simulink model "sistema_completo_con_controlador_pid_no_ideal"  (R2019a)
settings: Solver=VariableStepAuto  StartTime=0.0  StopTime=25  MaxStep=1e-5  RelTol=1e-5
undefined symbols (not defined in the file): A_sensor_curr, A_sensor_pos, A_sensor_temp, alpha_cu, b_eq, B_sensor_curr, B_sensor_pos, B_sensor_temp, C_sensor_curr, C_sensor_pos, C_sensor_temp, C_ts, D_sensor_curr, D_sensor_pos, D_sensor_temp, dT_l, J_eq, K_d, K_i, K_p, Ke_theta, Ke_w, L_d, L_ls, L_q, lambda_m, P_p, r, R_0, R_d, R_q, R_s_40, R_ts_amb, t_high, t_rise, w_max
libraries: eeTransforms x5, simulink x3
settings Model: Creator=pedro  LastModifiedBy=pedro

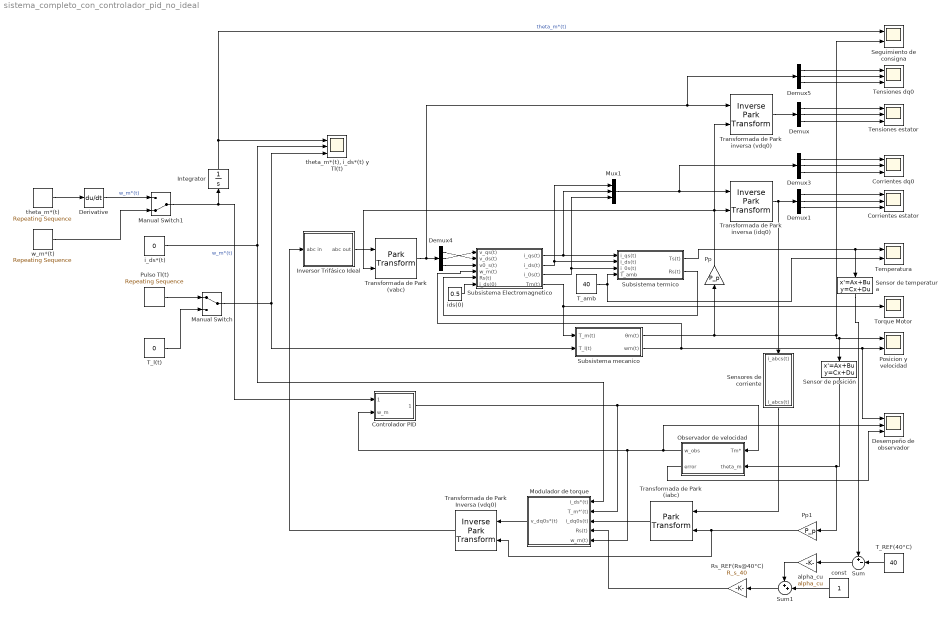
== system sistema_completo_con_controlador_pid_no_ideal ==
  " theta_m*(t), i_ds*(t) y Tl(t)" : Scope  NumInputPorts=3
  Controlador PID : Subsystem
  Corrientes estator : Scope  NumInputPorts=3
  Corrientes dq0 : Scope  NumInputPorts=3
  Demux{,1,3..5} (5 alike) : Demux  Outputs=3
  Derivative : Derivative
  Desempeño de observador : Scope  NumInputPorts=3
  Integrator : Integrator
  Inversor Trifásico Ideal : Subsystem
  Manual Switch : ManualSwitch
  Manual Switch1 : ManualSwitch  CurrentSetting=0
  Modulador de torque : Subsystem
  Mux1 : Mux  Inputs=3
  Observador de velocidad : Subsystem
  Posicion y velocidad : Scope  NumInputPorts=2
  Pp : Gain  Gain=P_p
  Pp1 : Gain  Gain=P_p
  Pulso Tl(t) : simulink/Sources/Repeating Sequence  rep_seq_t=[0 2.99 3 6.99 7 13.99 14 15.99 16 25]  rep_seq_y=[0 0 dT_l dT_l 0 0 -dT_l -dT_l 0 0]
  Rs_REF(Rs@40°C) : Gain  Gain=R_s_40
  Seguimiento de consigna : Scope  NumInputPorts=2
  Sensor de posición : StateSpace  A=A_sensor_pos  B=B_sensor_pos  C=C_sensor_pos  D=D_sensor_pos  InitialCondition=0  ContinuousStateAttributes="\"position\""
  Sensor de temperatura : StateSpace  A=A_sensor_temp  B=B_sensor_temp  C=C_sensor_temp  D=D_sensor_temp  InitialCondition=0  ContinuousStateAttributes="\"temperature\""
  Sensores de corriente : Subsystem
  Subsistema Electromagnetico : Subsystem
  "Subsistema mecanico " : Subsystem
  "Subsistema termico " : Subsystem
  Sum : Sum  Inputs=+-|
  Sum1 : Sum  Inputs=++|
  T_REF(40°C) : Constant  Value=40
  T_amb : Constant  Value=40
  T_l(t) : Constant  Value=0
  Temperatura : Scope  NumInputPorts=2
  Tensiones estator : Scope  NumInputPorts=3
  Tensiones dq0 : Scope  NumInputPorts=3
  Torque Motor : Scope
  Transformada de Park (iabc) : eeTransforms/Park Transform  AxisAlignment=Q-axis  PowerInvariant=off
      settings: SourceProductName=Simscape Electrical
  "Transformada de Park (vabc) " : eeTransforms/Park Transform  AxisAlignment=Q-axis  PowerInvariant=off
      settings: SourceProductName=Simscape Electrical
  Transformada de Park Inversa (vdq0) : eeTransforms/Inverse Park Transform  AxisAlignment=Q-axis  PowerInvariant=off
      settings: SourceProductName=Simscape Electrical
  Transformada de Park inversa (idq0) : eeTransforms/Inverse Park Transform  AxisAlignment=Q-axis  PowerInvariant=off
      settings: SourceProductName=Simscape Electrical
  "Transformada de Park inversa (vdq0) " : eeTransforms/Inverse Park Transform  AxisAlignment=Q-axis  PowerInvariant=off
      settings: SourceProductName=Simscape Electrical
  alpha_cu : Gain  Gain=alpha_cu
  const : Constant
  i_ds*(t) : Constant  Value=0
  ids(0) : Constant  Value=0.5
  theta_m*(t) : simulink/Sources/Repeating Sequence  rep_seq_t=[0 5 10 15 20 25]  rep_seq_y=[0 0 2*r*pi 2*r*pi 0 0]
  w_m*(t) : simulink/Sources/Repeating Sequence  rep_seq_t=[0 5 (5+t_rise) (5+t_rise+t_high) (5+2*t_rise+t_high) 15 (15+t_rise) (15+t_rise+t_high) (15+2*t_rise+t_high) 25]  rep_seq_y=[0 0 w_max w_max 0 0 -w_max -w_max 0 0]
  wires:
  Subsistema Electromagnetico/1("i_qs(t) ") -> Mux1/2, "Subsistema termico "/1("i_qs(t) ")
  Pp1/1 -> Transformada de Park Inversa (vdq0)/2, Transformada de Park (iabc)/2
  ids(0)/1 -> Subsistema Electromagnetico/6(i_ds(0))
  Demux/1 -> Tensiones estator/1
  Demux3/2 -> Corrientes dq0/2
  Transformada de Park inversa (idq0)/1 -> Demux1/1, Sensores de corriente/1(i_abcs(t))
  Sensores de corriente/1("i_abcs(t) ") -> Transformada de Park (iabc)/1
  Demux1/3 -> Corrientes estator/3
  Demux5/2 -> Tensiones dq0/2
  Demux/3 -> Tensiones estator/3
  Demux5/3 -> Tensiones dq0/3
  Demux/2 -> Tensiones estator/2
  Demux4/3 -> Subsistema Electromagnetico/3(v0_s(t))
  Inversor Trifásico Ideal/1(abc out) -> "Transformada de Park (vabc) "/1
  "Subsistema termico "/2(Rs(t)) -> Subsistema Electromagnetico/5("Rs(t) ")
  Pp/1 -> "Transformada de Park (vabc) "/2, Transformada de Park inversa (idq0)/2, "Transformada de Park inversa (vdq0) "/2
  Manual Switch/1 -> " theta_m*(t), i_ds*(t) y Tl(t)"/3, "Subsistema mecanico "/2("T_l(t) ")
  Demux1/2 -> Corrientes estator/2
  Demux4/2 -> Subsistema Electromagnetico/1(v_qs(t))
  Subsistema Electromagnetico/3("i_0s(t) ") -> Mux1/3, "Subsistema termico "/3(i_0s(t))
  "Transformada de Park inversa (vdq0) "/1 -> Demux/1
  Demux4/1 -> Subsistema Electromagnetico/2(v_ds(t))
  T_amb/1 -> Temperatura/2, "Subsistema termico "/4(T_amb)
  Demux1/1 -> Corrientes estator/1
  "Transformada de Park (vabc) "/1 -> Demux5/1, "Transformada de Park inversa (vdq0) "/1, Demux4/1
  Demux5/1 -> Tensiones dq0/1
  Transformada de Park (iabc)/1 -> Modulador de torque/3(i_dq0s(t))
  Demux3/3 -> Corrientes dq0/3
  Demux3/1 -> Corrientes dq0/1
  Mux1/1 -> Transformada de Park inversa (idq0)/1, Demux3/1
  Subsistema Electromagnetico/2(i_ds(t)) -> Mux1/1, "Subsistema termico "/2("i_ds(t) ")
  "Subsistema mecanico "/2(wm(t)) -> Posicion y velocidad/2, Desempeño de observador/1, Subsistema Electromagnetico/4(w_m(t))
  "Subsistema mecanico "/1(θm(t)) -> Sensor de posición/1, Posicion y velocidad/1, Seguimiento de consigna/2, Pp/1
  Subsistema Electromagnetico/4(Tm(t)) -> "Subsistema mecanico "/1("T_m(t) "), Torque Motor/1
  "Subsistema termico "/1(Ts(t)) -> Temperatura/1, Sensor de temperatura/1
  Sensor de posición/1 -> Pp1/1, Observador de velocidad/2(theta_m)
  Transformada de Park Inversa (vdq0)/1 -> Inversor Trifásico Ideal/1(abc in)
  i_ds*(t)/1 -> Modulador de torque/1(i_ds*(t)), " theta_m*(t), i_ds*(t) y Tl(t)"/2
  Observador de velocidad/1(w_obs) -> Desempeño de observador/2, Modulador de torque/5(w_m(t)), Controlador PID/2(w_m)
  Controlador PID/1(T_m*'(t)) -> Modulador de torque/2(T_m*'(t)), Observador de velocidad/1(Tm*)
  Modulador de torque/1(v_dq0s*(t)) -> Transformada de Park Inversa (vdq0)/1
  theta_m*(t)/1 -> Derivative/1
  Manual Switch1/1 -> Integrator/1, Controlador PID/1(w_m*)  "w_m*(t)"
  Observador de velocidad/2(error) -> Desempeño de observador/3
  Pulso Tl(t)/1 -> Manual Switch/1
  T_l(t)/1 -> Manual Switch/2
  Derivative/1 -> Manual Switch1/1  "w_m*(t)"
  Integrator/1 -> " theta_m*(t), i_ds*(t) y Tl(t)"/1, Seguimiento de consigna/1  "theta_m*(t)"
  w_m*(t)/1 -> Manual Switch1/2
  Sum/1 -> alpha_cu/1
  alpha_cu/1 -> Sum1/1
  Sum1/1 -> Rs_REF(Rs@40°C)/1
  const/1 -> Sum1/2
  T_REF(40°C)/1 -> Sum/2
  Sensor de temperatura/1 -> Sum/1
  Rs_REF(Rs@40°C)/1 -> Modulador de torque/4(Rs(t))

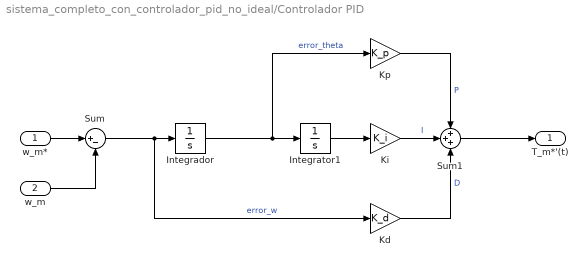
== system sistema_completo_con_controlador_pid_no_ideal/Controlador PID ==
  w_m* : Inport
  w_m : Inport  Port=2
  Integrador : Integrator
  Integrator1 : Integrator
  Kd : Gain  Gain=K_d
  Ki : Gain  Gain=K_i
  Kp : Gain  Gain=K_p
  Sum : Sum  Inputs=|+-
  Sum1 : Sum  Inputs=+++
  T_m*'(t) : Outport
  wires:
  Sum/1 -> Kd/1, Integrador/1  "error_w"
  w_m/1 -> Sum/2
  Sum1/1 -> T_m*'(t)/1
  Integrador/1 -> Integrator1/1, Kp/1  "error_theta"
  Kd/1 -> Sum1/3  "D"
  Integrator1/1 -> Ki/1
  w_m*/1 -> Sum/1
  Ki/1 -> Sum1/2  "I"
  Kp/1 -> Sum1/1  "P"

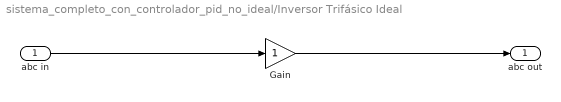
== system sistema_completo_con_controlador_pid_no_ideal/Inversor Trifásico Ideal ==
  abc in : Inport
  Gain : Gain
  abc out : Outport
  wires:
  abc in/1 -> Gain/1
  Gain/1 -> abc out/1

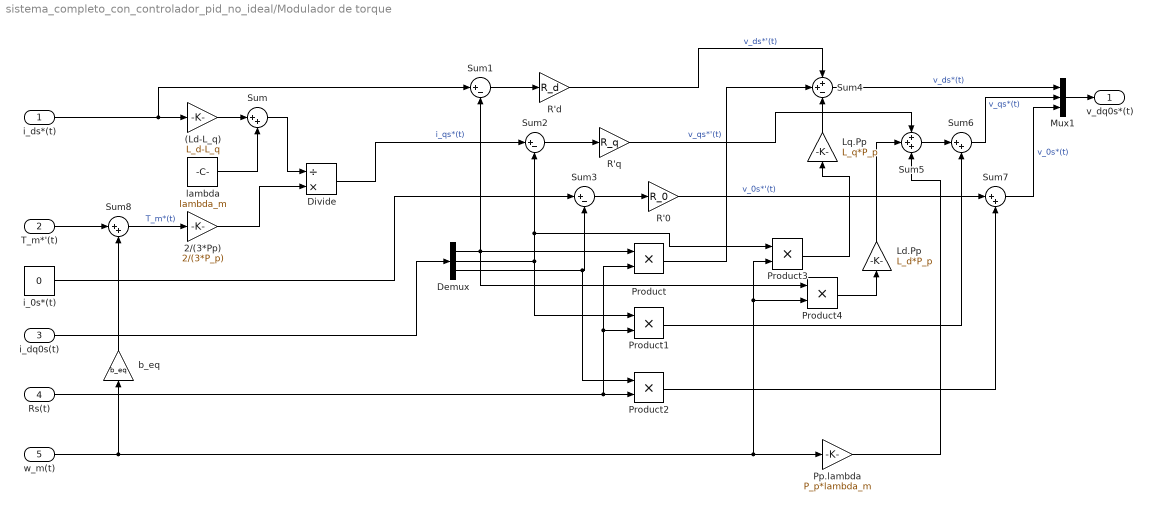
== system sistema_completo_con_controlador_pid_no_ideal/Modulador de torque ==
  i_ds*(t) : Inport
  T_m*'(t) : Inport  Port=2
  i_dq0s(t) : Inport  Port=3
  Rs(t) : Inport  Port=4
  w_m(t) : Inport  Port=5
  (Ld-L_q) : Gain  Gain=L_d-L_q
  2/(3*Pp) : Gain  Gain=2/(3*P_p)
  Demux : Demux  Outputs=3
  Divide : Product  Inputs=/*
  Ld.Pp : Gain  Gain=L_d*P_p
  Lq.Pp : Gain  Gain=L_q*P_p
  Mux1 : Mux  Inputs=3
  Pp.lambda : Gain  Gain=P_p*lambda_m
  Product{,1..4} (5 alike) : Product
  R'0 : Gain  Gain=R_0
  R'd : Gain  Gain=R_d
  R'q : Gain  Gain=R_q
  Sum{,6..8} (4 alike) : Sum  Inputs=|++
  Sum1 : Sum  Inputs=|+-
  Sum2 : Sum  Inputs=|+-
  Sum3 : Sum  Inputs=|+-
  Sum4 : Sum  Inputs=++-
  Sum5 : Sum  Inputs=+++
  b_eq : Gain  Gain=b_eq
  i_0s*(t) : Constant  Value=0
  lambda : Constant  Value=lambda_m
  v_dq0s*(t) : Outport
  wires:
  lambda/1 -> Sum/2
  (Ld-L_q)/1 -> Sum/1
  Sum/1 -> Divide/1
  2/(3*Pp)/1 -> Divide/2
  Divide/1 -> Sum2/1  "i_qs*(t)"
  Mux1/1 -> v_dq0s*(t)/1
  Product4/1 -> Ld.Pp/1
  R'0/1 -> Sum7/1  "v_0s*'(t)"
  Sum5/1 -> Sum6/1
  Sum6/1 -> Mux1/2  "v_qs*(t)"
  Product1/1 -> Sum6/2
  Sum2/1 -> R'q/1
  Sum7/1 -> Mux1/3  "v_0s*(t)"
  Lq.Pp/1 -> Sum4/3
  Product/1 -> Sum4/2
  Demux/2 -> Product3/1, Sum2/2, Product1/1
  Product2/1 -> Sum7/2
  Sum4/1 -> Mux1/1  "v_ds*(t)"
  Pp.lambda/1 -> Sum5/3
  R'd/1 -> Sum4/1  "v_ds*'(t)"
  Demux/1 -> Product4/1, Product/1, Sum1/2
  Sum3/1 -> R'0/1
  i_0s*(t)/1 -> Sum3/1
  Rs(t)/1 -> Product1/2, Product/2, Product2/2
  w_m(t)/1 -> Product3/2, Product4/2, Pp.lambda/1, b_eq/1
  Ld.Pp/1 -> Sum5/2
  R'q/1 -> Sum5/1  "v_qs*'(t)"
  Product3/1 -> Lq.Pp/1
  Demux/3 -> Product2/1, Sum3/2
  i_ds*(t)/1 -> Sum1/1, (Ld-L_q)/1
  Sum1/1 -> R'd/1
  i_dq0s(t)/1 -> Demux/1
  b_eq/1 -> Sum8/2
  T_m*'(t)/1 -> Sum8/1
  Sum8/1 -> 2/(3*Pp)/1  "T_m*(t)"

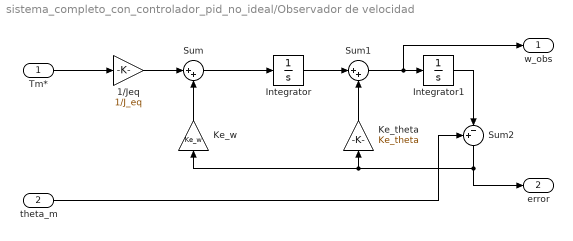
== system sistema_completo_con_controlador_pid_no_ideal/Observador de velocidad ==
  Tm* : Inport
  theta_m : Inport  Port=2
  1/Jeq : Gain  Gain=1/J_eq
  Integrator : Integrator
  Integrator1 : Integrator
  Ke_theta : Gain  Gain=Ke_theta
  Ke_w : Gain  Gain=Ke_w
  Sum : Sum  Inputs=|++
  Sum1 : Sum  Inputs=|++
  Sum2 : Sum  Inputs=+-|
  w_obs : Outport
  error : Outport  Port=2
  wires:
  Integrator/1 -> Sum1/1
  Sum1/1 -> w_obs/1, Integrator1/1
  Sum2/1 -> error/1, Ke_w/1, Ke_theta/1
  Integrator1/1 -> Sum2/2
  Ke_w/1 -> Sum/2
  Tm*/1 -> 1/Jeq/1
  1/Jeq/1 -> Sum/1
  Sum/1 -> Integrator/1
  Ke_theta/1 -> Sum1/2
  theta_m/1 -> Sum2/1

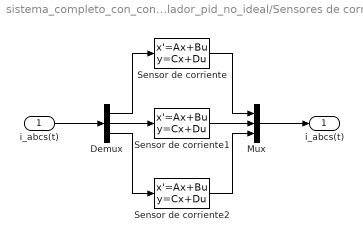
== system sistema_completo_con_controlador_pid_no_ideal/Sensores de corriente ==
  i_abcs(t) : Inport
  Demux : Demux  Outputs=3
  Mux : Mux  Inputs=3
  Sensor de corriente : StateSpace  A=A_sensor_curr  B=B_sensor_curr  C=C_sensor_curr  D=D_sensor_curr  InitialCondition=0  ContinuousStateAttributes="\"current\""
  Sensor de corriente1 : StateSpace  A=A_sensor_curr  B=B_sensor_curr  C=C_sensor_curr  D=D_sensor_curr  InitialCondition=0  ContinuousStateAttributes="\"current\""
  Sensor de corriente2 : StateSpace  A=A_sensor_curr  B=B_sensor_curr  C=C_sensor_curr  D=D_sensor_curr  InitialCondition=0  ContinuousStateAttributes="\"current\""
  "i_abcs(t) " : Outport
  wires:
  Demux/2 -> Sensor de corriente1/1
  Sensor de corriente1/1 -> Mux/2
  Mux/1 -> "i_abcs(t) "/1
  i_abcs(t)/1 -> Demux/1
  Demux/1 -> Sensor de corriente/1
  Sensor de corriente/1 -> Mux/1
  Demux/3 -> Sensor de corriente2/1
  Sensor de corriente2/1 -> Mux/3

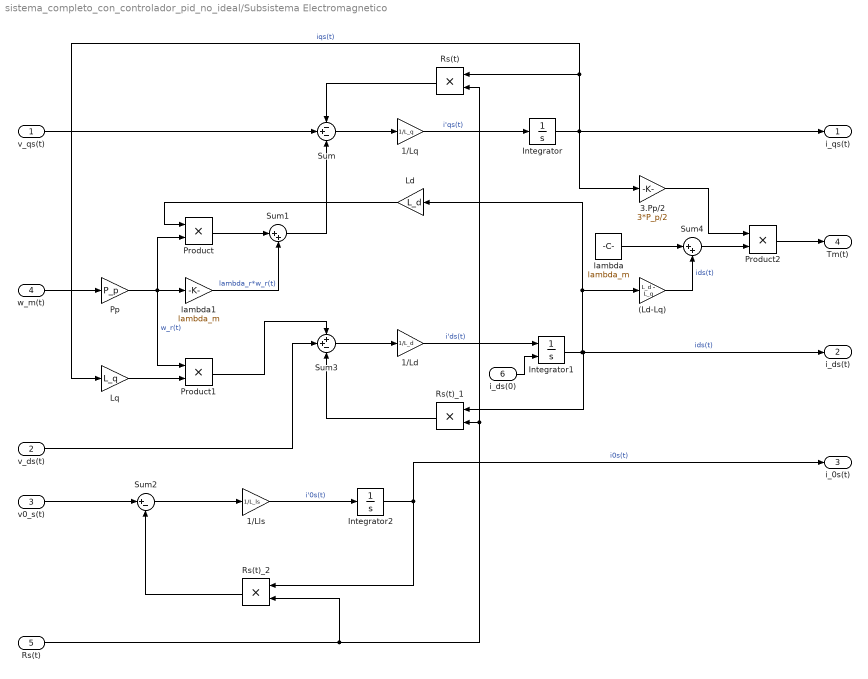
== system sistema_completo_con_controlador_pid_no_ideal/Subsistema Electromagnetico ==
  v_qs(t) : Inport
  v_ds(t) : Inport  Port=2
  v0_s(t) : Inport  Port=3
  w_m(t) : Inport  Port=4
  "Rs(t) " : Inport  Port=5
  i_ds(0) : Inport  Port=6
  (Ld-Lq) : Gain  Gain=L_d - L_q
  1/Ld : Gain  Gain=1/L_d
  1/Lls : Gain  Gain=1/L_ls
  1/Lq : Gain  Gain=1/L_q
  3.Pp/2 : Gain  Gain=3*P_p/2
  Integrator : Integrator
  Integrator1 : Integrator  InitialConditionSource=external
  Integrator2 : Integrator
  Ld : Gain  Gain=L_d
  Lq : Gain  Gain=L_q
  Pp : Gain  Gain=P_p
  Product : Product
  Product1 : Product
  Product2 : Product
  Rs(t) : Product
  Rs(t)_1 : Product
  Rs(t)_2 : Product
  Sum : Sum  Inputs=-+-
  Sum1 : Sum  Inputs=|++
  Sum2 : Sum  Inputs=|+-
  Sum3 : Sum  Inputs=++-
  Sum4 : Sum  Inputs=|++
  lambda : Constant  Value=lambda_m
  lambda1 : Gain  Gain=lambda_m
  "i_qs(t) " : Outport
  i_ds(t) : Outport  Port=2
  "i_0s(t) " : Outport  Port=3
  Tm(t) : Outport  Port=4
  wires:
  w_m(t)/1 -> Pp/1
  Pp/1 -> Product1/1, Product/2, lambda1/1  "w_r(t)"
  Sum/1 -> 1/Lq/1
  1/Lq/1 -> Integrator/1  "i'qs(t)"
  Sum1/1 -> Sum/3
  v_qs(t)/1 -> Sum/2
  Integrator/1 -> Lq/1, Rs(t)/1, 3.Pp/2/1, "i_qs(t) "/1  "iqs(t)"
  lambda1/1 -> Sum1/2  "lambda_r*w_r(t)"
  Product/1 -> Sum1/1
  v_ds(t)/1 -> Sum3/2
  Sum3/1 -> 1/Ld/1
  Product1/1 -> Sum3/1
  1/Ld/1 -> Integrator1/1  "i'ds(t)"
  Integrator1/1 -> Ld/1, (Ld-Lq)/1, Rs(t)_1/1, i_ds(t)/1  "ids(t)"
  Lq/1 -> Product1/2
  Ld/1 -> Product/1
  v0_s(t)/1 -> Sum2/1
  Rs(t)_2/1 -> Sum2/2
  Sum2/1 -> 1/Lls/1
  1/Lls/1 -> Integrator2/1  "i'0s(t)"
  Integrator2/1 -> Rs(t)_2/1, "i_0s(t) "/1  "i0s(t)"
  (Ld-Lq)/1 -> Sum4/2  "ids(t)"
  lambda/1 -> Sum4/1
  Sum4/1 -> Product2/2
  Product2/1 -> Tm(t)/1
  3.Pp/2/1 -> Product2/1
  "Rs(t) "/1 -> Rs(t)_2/2, Rs(t)/2, Rs(t)_1/2
  Rs(t)_1/1 -> Sum3/3
  Rs(t)/1 -> Sum/1
  i_ds(0)/1 -> Integrator1/2

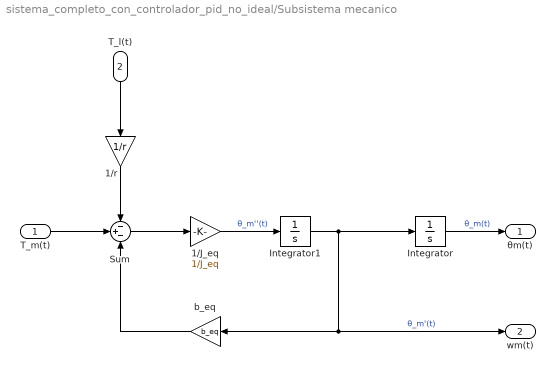
== system sistema_completo_con_controlador_pid_no_ideal/Subsistema mecanico  ==
  "T_m(t) " : Inport
  "T_l(t) " : Inport  Port=2
  "1/J_eq " : Gain  Gain=1/J_eq
  1/r : Gain  Gain=1/r
  Integrator : Integrator
  Integrator1 : Integrator
  Sum : Sum  Inputs=-+-
  b_eq : Gain  Gain=b_eq
  θm(t) : Outport
  wm(t) : Outport  Port=2
  wires:
  Integrator1/1 -> b_eq/1, wm(t)/1, Integrator/1  "θ_m'(t)"
  Sum/1 -> "1/J_eq "/1
  b_eq/1 -> Sum/3
  "1/J_eq "/1 -> Integrator1/1  "θ_m''(t)"
  Integrator/1 -> θm(t)/1  "θ_m(t)"
  "T_m(t) "/1 -> Sum/2
  "T_l(t) "/1 -> 1/r/1
  1/r/1 -> Sum/1

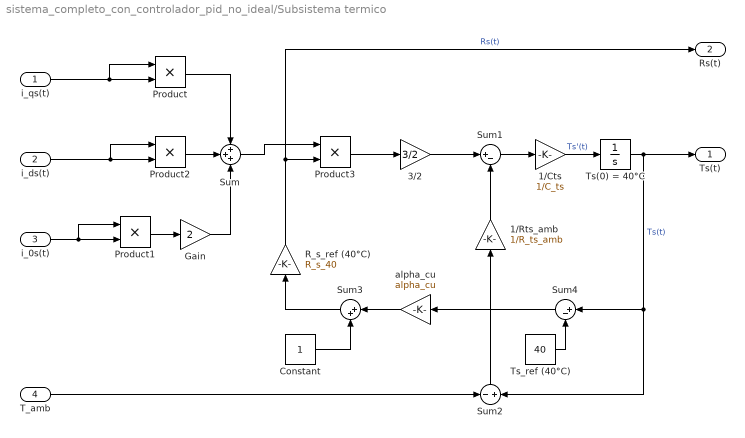
== system sistema_completo_con_controlador_pid_no_ideal/Subsistema termico  ==
  "i_qs(t) " : Inport
  "i_ds(t) " : Inport  Port=2
  i_0s(t) : Inport  Port=3
  T_amb : Inport  Port=4
  1/Cts : Gain  Gain=1/C_ts
  1/Rts_amb : Gain  Gain=1/R_ts_amb
  3/2 : Gain  Gain=3/2
  Constant : Constant
  Gain : Gain  Gain=2
  Product{,1..3} (4 alike) : Product
  R_s_ref (40°C) : Gain  Gain=R_s_40
  Sum : Sum  Inputs=+++
  Sum1 : Sum  Inputs=|+-
  Sum2 : Sum  Inputs=-|+
  Sum3 : Sum  Inputs=|++
  Sum4 : Sum  Inputs=|+-
  Ts(0) = 40°C : Integrator  InitialCondition=40
  Ts_ref (40°C) : Constant  Value=40
  alpha_cu : Gain  Gain=alpha_cu
  Ts(t) : Outport
  Rs(t) : Outport  Port=2
  wires:
  i_0s(t)/1 -> Product1/1, Product1/2
  "i_ds(t) "/1 -> Product2/1, Product2/2
  "i_qs(t) "/1 -> Product/1, Product/2
  Product/1 -> Sum/1
  Product2/1 -> Sum/2
  Ts(0) = 40°C/1 -> Sum4/1, Sum2/2, Ts(t)/1  "Ts(t)"
  T_amb/1 -> Sum2/1
  Sum2/1 -> 1/Rts_amb/1
  1/Rts_amb/1 -> Sum1/2
  Sum1/1 -> 1/Cts/1
  1/Cts/1 -> Ts(0) = 40°C/1  "Ts'(t)"
  Constant/1 -> Sum3/2
  alpha_cu/1 -> Sum3/1
  Sum3/1 -> R_s_ref (40°C)/1
  R_s_ref (40°C)/1 -> Rs(t)/1, Product3/2  "Rs(t)"
  Sum/1 -> Product3/1
  Product3/1 -> 3/2/1
  3/2/1 -> Sum1/1
  Ts_ref (40°C)/1 -> Sum4/2
  Sum4/1 -> alpha_cu/1
  Gain/1 -> Sum/3
  Product1/1 -> Gain/1
